simulink model "gm_MVB3sender"  (R2013b)
settings: Solver=FixedStepDiscrete  SolverMode=SingleTasking  StartTime=0  StopTime=8000  RelTol=1e-3
model workspace (MAT data in the model file):
  logicAddr = 2
settings Model: Creator=qiji  LastModifiedBy=qiji
settings OptimizationCC: BlockReduction=off  ConditionallyExecuteInputs=off  InlineParams=on
settings DebuggingCC: UnderspecifiedInitializationDetection=Simplified  MultiTaskDSMMsg=warning  MultiTaskCondExecSysMsg=none  SingleTaskRateTransMsg=error  SFUnusedDataAndEventsDiag=none
settings RTWCC: IncludeERTFirstTime=on
settings GRTTargetCC: CodeReplacementLibrary=None  CPPClassGenCompliant=on
settings ConfigurationSet: Description=SimMechanics 2G

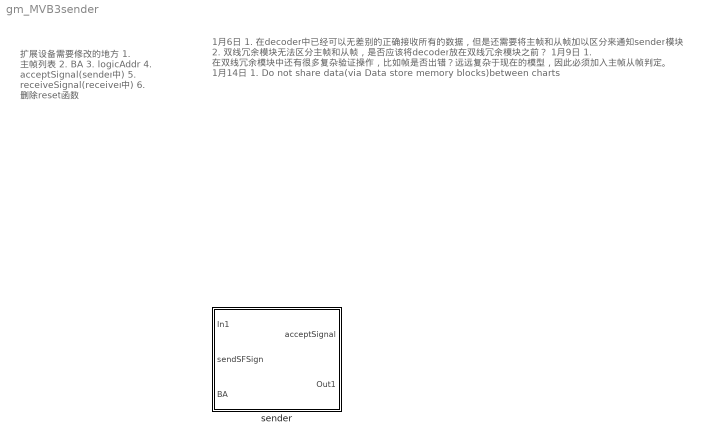
== system gm_MVB3sender ==
  note: 1月6日
      | 1. 在decoder中已经可以无差别的正确接收所有的数据，但是还需要将主帧和从帧加以区分来通知sender模块
      | 2. 双线冗余模块无法区分主帧和从帧，是否应该将decoder放在双线冗余模块之前？
      | 1月9日
      | 1. 在双线冗余模块中还有很多复杂验证操作，比如帧是否出错？远远复杂于现在的模型，因此必须加入主帧从帧判定。
      | 1月14日
      | 1. Do not share data(via Data store memory blocks)between charts
  note: 扩展设备需要修改的地方
      | 1. 主帧列表
      | 2. BA
      | 3. logicAddr
      | 4. acceptSignal(sender中)
      | 5. receiveSignal(receiver中)
      | 6. 删除reset函数
  sender : Subsystem

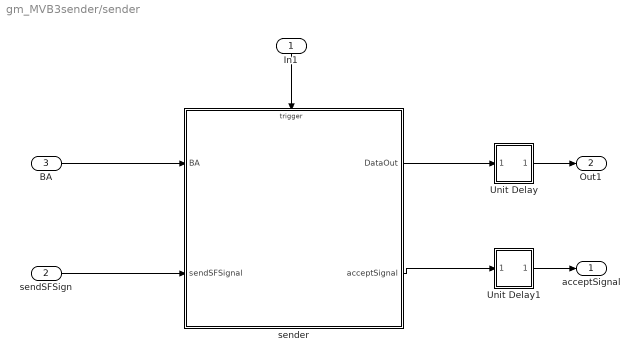
== system gm_MVB3sender/sender ==
  In1 : Inport  OutDataTypeStr=boolean
  sendSFSign : Inport  Port=2
  BA : Inport  Port=3
  Unit Delay : Subsystem
  Unit Delay1 : Subsystem
  sender : Stateflow chart  TreatAsAtomicUnit=on
  acceptSignal : Outport
  Out1 : Outport  Port=2
  wires:
  Unit Delay1/1(Out) -> acceptSignal/1
  BA/1 -> sender/1(BA)
  sender/2(acceptSignal) -> Unit Delay1/1(In1)
  sendSFSign/1 -> sender/2(sendSFSignal)
  In1/1 -> sender/Trigger
  sender/1(DataOut) -> Unit Delay/1(In1)
  Unit Delay/1(Out) -> Out1/1

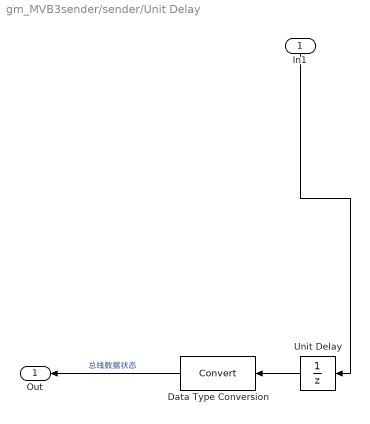
== system gm_MVB3sender/sender/Unit Delay ==
  In1 : Inport
  Data Type Conversion : DataTypeConversion
  Unit Delay : UnitDelay  SampleTime=-1
  Out : Outport
  wires:
  Data Type Conversion/1 -> Out/1  "总线数据状态"
  Unit Delay/1 -> Data Type Conversion/1
  In1/1 -> Unit Delay/1

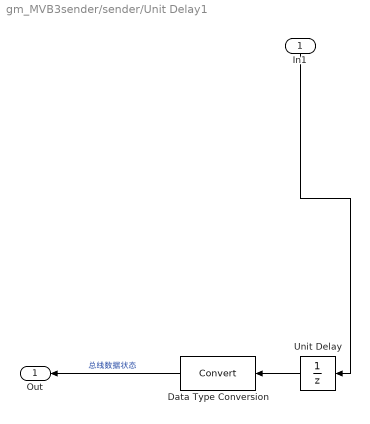
== system gm_MVB3sender/sender/Unit Delay1 ==
  In1 : Inport
  Data Type Conversion : DataTypeConversion
  Unit Delay : UnitDelay  SampleTime=-1
  Out : Outport
  wires:
  In1/1 -> Unit Delay/1
  Unit Delay/1 -> Data Type Conversion/1
  Data Type Conversion/1 -> Out/1  "总线数据状态"

== stateflow chart gm_MVB3sender/sender/sender ==
  settings: executeAtInitialization=1  initializeOutput=1
  state SFSender [parallel]
    settings: executionOrder=1
    note: send**Signd的置位在接收到了请求数据的主帧后置位
    state sender [parallel]
      settings: executionOrder=1
      state wait
      state sendRandomSF
      state sendOK
      state sendInfo
      state transmission
        en:
        enterTrans = true;
        ex:
        enterTrans = false;
      (default) -> SFSender.sender.wait
      SFSender.sender.wait -> sendRandomSF [order 1] : [sendSFSignal==1]
      SFSender.sender.wait -> sendInfo [order 3] : [ sendSFSignal==2]
      SFSender.sender.wait -> sendOK [order 2] : [sendSFSignal==3]
      sendRandomSF -> SFSender.sender.transmission : {SFIndex = uint8(0);}
      sendOK -> SFSender.sender.transmission : {SFIndex = uint8(2);
          | init();
          | }
      sendInfo -> SFSender.sender.transmission : {SFIndex = uint8(1);}
      SFSender.sender.transmission -> SFSender.sender : [SFTransDone == true]
          | {DataOut = uint32(0);}
          | /{SFTransDone = false;}
    state sendHolder [parallel]
      settings: executionOrder=2
      state judge
      state full
        SFSender.sendHolder.full -> SFSender.sendHolder.full [order 1] : CLK
            | {
            | DataOut = bitoperate.getbit(input);
            | input = bitoperate.shiftbit(input, uint32(1));
            | count = count + uint8(1);
            | }
      state empty
      SFSender.sendHolder.judge -> SFSender.sendHolder.empty [order 2] : {
          | SFCurrentIndex = uint8(2);
          | SFTransDone = true;
          | }
      SFSender.sendHolder.full -> SFSender.sendHolder.judge [order 1] : [count == uint8(32)]
          | {
          | SFCurrentIndex = SFCurrentIndex + uint8(1);
          | }
      SFSender.sendHolder.judge -> SFSender.sendHolder.full [order 1] : [SFCurrentIndex <= SFT[SFIndex*16 + 1]]
          | {
          | input = ManchesterEncoding(uint32(SFT[SFIndex*16+SFCurrentIndex]));
          | count = uint8(0);
          | }
      (default) -> SFSender.sendHolder.empty : {
          | SFCurrentIndex = uint8(2);
          | SFTransDone = false;
          | }
      SFSender.sendHolder.empty -> SFSender.sendHolder.full : [enterTrans == true]
          | {
          | input = ManchesterEncoding(uint32(SFT[SFIndex*16+SFCurrentIndex]));
          | DataOut = uint32(0);
          | count = uint8(0);
          | }
  state MFSender [parallel]
    settings: executionOrder=2
    state sender [parallel]
      settings: executionOrder=2
      state transmission
        en:
        enterTrans = true;
        acceptSignal =setAcceptSignal(MFT[MFIndex*16+3]);
        ex:
        enterTrans = false;
      state sleep
      state wait
      (default) -> sleep : {
          | init();
          | }
      MFSender.sender.transmission -> sleep : [MFTransDone==true]
          | {
          | DataOut = uint32(0);
          | MFIndex = MFIndex + uint8(1);
          | MFTransDone=false;
          | }
      sleep -> MFSender.sender.wait : every(150, CLK)
          | [master==true]
      MFSender.sender.wait -> MFSender.sender.transmission
    state sendHolder [parallel]
      settings: executionOrder=3
      state judge
      state full
        MFSender.sendHolder.full -> MFSender.sendHolder.full [order 1] : CLK
            | {
            | DataOut = bitoperate.getbit(input);
            | input = bitoperate.shiftbit(input, uint32(1));
            | count = count + uint8(1);
            | }
      state empty
      MFSender.sendHolder.judge -> MFSender.sendHolder.empty [order 2] : {
          | MFCurrentIndex = uint8(2);
          | MFTransDone=true;
          | }
      MFSender.sendHolder.full -> MFSender.sendHolder.judge [order 1] : [count == uint8(32)]
          | {
          | MFCurrentIndex = MFCurrentIndex + uint8(1);
          | }
      MFSender.sendHolder.judge -> MFSender.sendHolder.full [order 1] : [MFCurrentIndex <= MFT[MFIndex*16 + 1]]
          | {
          | input =ManchesterEncoding(uint32(MFT[MFIndex*16+MFCurrentIndex]));
          | count = uint8(0);
          | }
      (default) -> MFSender.sendHolder.empty : {
          | MFCurrentIndex = uint8(2);
          | MFTransDone=false;
          | }
      MFSender.sendHolder.empty -> MFSender.sendHolder.full : [enterTrans == true]
          | {
          | input = ManchesterEncoding(uint32(MFT[MFIndex*16+MFCurrentIndex]));
          | DataOut = uint32(0);
          | count = uint8(0);
          | }
    state BAHolder [parallel]
      settings: executionOrder=1
      state false
        du:
        master = false;
      state true
        du:
        master = true;
      false -> true : [BA == true]
          | {master = true;}
      (default) -> true
      true -> false : [BA == true]
          | {master =false;}
  state init [function]
    note: F_code=0
        | addr=2
        | 0010//1100/0111/0001
        | 0101//0000/0000/0000
        | 0010//1010/1000/1110
        | 0000/0000/0011//0011
        | F_code=8
        | addr=2
        | 0010//1100/0111/0001
        | 0101//1000/0000/0000
        | 0010//1010/1000/1110
        | 0000/0000/0011//0011
        | F_code=0
        | addr=2
        | 0010//1100/0111/0001
        | 0101//1111/0000/0000
        | 0010//1010/1000/1110
        | 0000/0000/0011//0011
    note: 请求随机从帧
        | 请求随机从帧
        | 请求2号的信息
        | 请求转移到2号
    note: SFT(1)代表随机的从帧
        | SFT(2)代表回复接受主权
        | SFT(3)代表回复设备ACT和BA
    (default) -> (junction 77) : {
        | MFIndex = uint8(0);
        | acceptSignal = uint8(0);
        | MFT[1] = uint16(5);
        | MFT[2] = uint16(11377);
        | MFT[3] = uint16(20480);
        | MFT[4] = uint16(10894);
        | MFT[5] = uint16(51);
        |
        | MFT[17] = uint16(5);
        | MFT[18] = uint16(11377);
        | MFT[19] = uint16(20480);
        | MFT[20] = uint16(14990);
        | MFT[21] = uint16(51);
        |
        | MFT[33] = uint16(5);
        | MFT[34] = uint16(11377);
        | MFT[35] = uint16(22528);
        | MFT[36] = uint16(10894);
        | MFT[37] = uint16(51);
        |
        | MFT[49] = uint16(5);
        | MFT[50] = uint16(11377);
        | MFT[51] = uint16(24320);
        | MFT[52] = uint16(10894);
        | MFT[53] = uint16(51);
        |
        |
        | SFT[1] = uint16(4);
        | SFT[2] = uint16(10894);
        | SFT[3] = uint16(12428);
        | SFT[4] = uint16(19);
        | SFT[17] = uint16(4);
        | SFT[18] = uint16(10894);
        | SFT[19] = uint16(12832);
        | SFT[20] = uint16(3);
        | SFT[33] = uint16(4);
        | SFT[34] = uint16(10894);
        | SFT[35] = uint16(14464);
        | SFT[36] = uint16(3);
        | }
  state bitoperate [group]
  note: MFT(1) = 5;
      | MFT(2) = 11377;
      | MFT(3) = 20480;
      | MFT(4) = 10894;
      | MFT(5) = 51;
      |
      | MFT(17) = 5;
      | MFT(18) = 11377;
      | MFT(19) = 20480;
      | MFT(20) = 10894;
      | MFT(21) = 51;
      |
      | MFT(33) = 5;
      | MFT(34) = 11377;
      | MFT(35) = 22528;
      | MFT(36) = 10894;
      | MFT(37) = 51;
      |
      | MFT(49) = 5
      | MFT(50) = 11377;
      | MFT(52) = 24320;
      | MFT(53) = 10894;
      | MFT(54) = 51;
  data: SFCurrentIndex local uint8; count local uint8; input local uint32; SFTransDone local boolean; SFIndex local uint8; enterTrans local boolean; data function_input uint16; Signal function_output uint8; bit1 temporary uint16; bit2 temporary uint16; bit3 temporary uint16; bit0 temporary uint16; i function_input double; r function_output uint8; MFCurrentIndex local uint8; count local uint8; input local uint32; MFTransDone local boolean; enterTrans local boolean; data function_input uint32; r function_output uint32; r function_output uint32; data function_input uint32; num function_input uint32; r function_output uint32; data function_input uint32; num function_input uint32; r function_output uint32; BA input boolean; sendSFSignal input uint8; MFT local uint16 size=100; SFT local uint16 size=100; DataOut output uint32; acceptSignal output uint8; MFIndex local uint8; master local boolean
  events: CLK input RISING_EDGE_EVENT
  function Signal = setAcceptSignal(data):
    | function Signal = setAcceptSignal(data)
    | bit0 = uint16(bitget(data, 9));
    | bit1 = uint16(bitget(data, 10));
    | bit2 = uint16(bitget(data, 11));
    | bit3 = uint16(bitget(data, 12));
    | fcode = bit0+bit1*2+bit2*4+bit3*8;
    | Signal=uint8(0);
    | if fcode==0
    |     Signal=uint8(1);
    | elseif fcode==8
    |     Signal=uint8(2);
    | elseif fcode==15
    |     Signal=uint8(3);
    | end
  function r = reset(i):
    | function r = reset(i)
    | if i==2
    |     r = uint8(0);
    | else
    |     r = uint8(i);
    | end
  function r = ManchesterEncoding(data):
    | function r = ManchesterEncoding(data)
    | r = data;
    | for i = 1:16
    |     x = bitget(data, i);
    |     if x == 0
    |         r = bitset(r, i*2-1, 1);
    |         r = bitset(r, i*2, 0);
    |     else
    |         r = bitset(r, i*2-1, 0);
    |         r = bitset(r, i*2, 1);
    |     end
    | end
  function r = ManchesterDecoding(data):
    | function r = ManchesterDecoding(data)
    | r = uint32(0);
    | for i = (1:2:32)
    |     x0 = bitget(data, i);
    |     x1 = bitget(data, i+1);
    |     if x0==0 && x1==1
    |         r = bitset(r, (i+1)/2, 1);
    |     else
    |         r = bitset(r, (i+1)/2, 0);
    |     end
    | end
  function r = getbit(num):
    | function r = getbit(num)
    | r = bitget(num, 32);
  function r = shiftbit(data, num):
    | function r = shiftbit(data, num)
    | r = bitshift(data, num);
    | %for i=1:cnt
    | %   r = bitset(r, i, 0);
    | %end
